simulink model "model6_3"  (R2024b)
settings: Solver=VariableStepAuto  StartTime=0.0  StopTime=100000  RelTol=1e-3
values from neighbouring files (symbols this model uses):
  Tf = 1    [domaci6_2.m]    (also in domaci6_3.m)
settings Model: Creator=neso  LastModifiedBy=neso

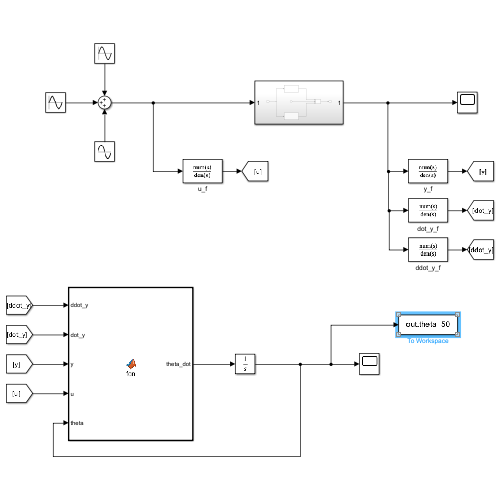
[thumbnail: Simulink's stored preview of the top-level diagram]
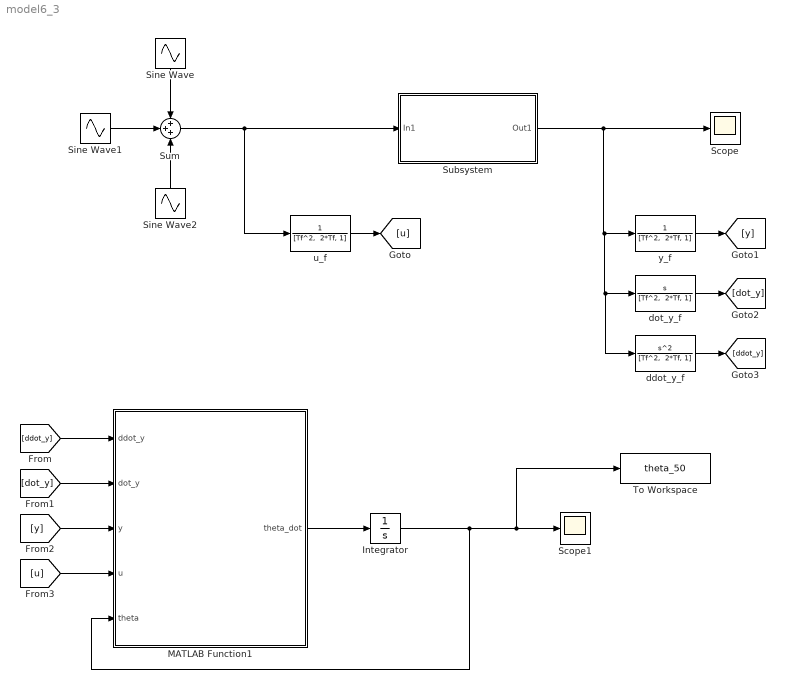
== system model6_3 ==
  Integrator : Integrator  InitialCondition=[0; 0; 0]
  MATLAB Function1 : MATLAB Function  TreatAsAtomicUnit=on
  Scope : Scope
  Scope1 : Scope
  Sine Wave : Sin  SampleTime=0
  Sine Wave1 : Sin  Frequency=2  SampleTime=0
  Sine Wave2 : Sin  Frequency=3  SampleTime=0
  Subsystem : Subsystem
  Sum : Sum  Inputs=+++
  To Workspace : ToWorkspace  VariableName=theta_50  SaveFormat=Timeseries  SampleTime=-1
  ddot_y_f : TransferFcn  Numerator=[1, 0, 0]  Denominator="[Tf^2,  2*Tf, 1]"
  dot_y_f : TransferFcn  Numerator=[1, 0]  Denominator="[Tf^2,  2*Tf, 1]"
  u_f : TransferFcn  Denominator="[Tf^2,  2*Tf, 1]"
  y_f : TransferFcn  Denominator="[Tf^2,  2*Tf, 1]"
  wires:
  u_f/1 -> [u]
  y_f/1 -> [y]
  dot_y_f/1 -> [dot_y]
  ddot_y_f/1 -> [ddot_y]
  MATLAB Function1/1(theta_dot) -> Integrator/1
  [ddot_y] -> MATLAB Function1/1(ddot_y)
  [dot_y] -> MATLAB Function1/2(dot_y)
  [y] -> MATLAB Function1/3(y)
  [u] -> MATLAB Function1/4(u)
  Integrator/1 -> To Workspace/1, Scope1/1, MATLAB Function1/5(theta)
  Sum/1 -> Subsystem/1(In1), u_f/1
  Sine Wave/1 -> Sum/1
  Sine Wave1/1 -> Sum/2
  Sine Wave2/1 -> Sum/3
  Subsystem/1(Out1) -> ddot_y_f/1, dot_y_f/1, y_f/1, Scope/1

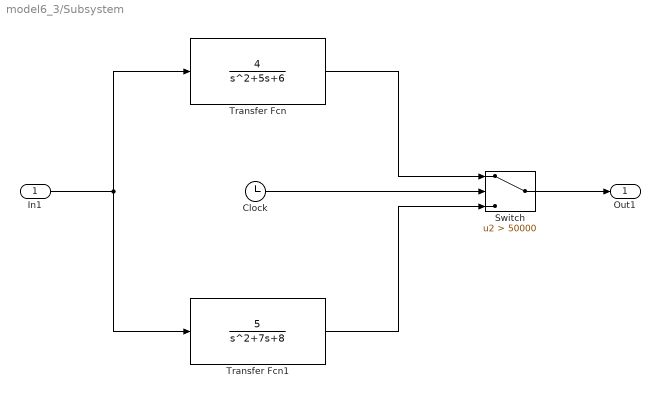
== system model6_3/Subsystem ==
  In1 : Inport
  Clock : Clock
  Switch : Switch  Criteria=u2 > Threshold  Threshold=50000  SaturateOnIntegerOverflow=off  InputSameDT=off
  Transfer Fcn : TransferFcn  Numerator=4  Denominator=[1, 5, 6]
  Transfer Fcn1 : TransferFcn  Numerator=5  Denominator=[1, 7, 8]
  Out1 : Outport
  wires:
  Clock/1 -> Switch/2
  In1/1 -> Transfer Fcn1/1, Transfer Fcn/1
  Transfer Fcn/1 -> Switch/1
  Transfer Fcn1/1 -> Switch/3
  Switch/1 -> Out1/1

== matlab function model6_3/MATLAB Function1 ==
  data: ddot_y input; dot_y input; y input; u input; theta_dot output; theta input
function theta_dot = fcn(ddot_y, dot_y, y, u, theta)
    p = [-dot_y; -y; u];
    eta = ddot_y;

    G = 50 * eye(length(p), length(p));

    theta_dot = G * p * (eta - p' * theta);
end
